simulink model "Problem_3"  (R2020a)
settings: Solver=VariableStepAuto  StartTime=0.0  StopTime=10.0  RelTol=1e-3
settings Model: Creator=Shubham Singh Rathor  LastModifiedBy=Shubham Singh Rathor

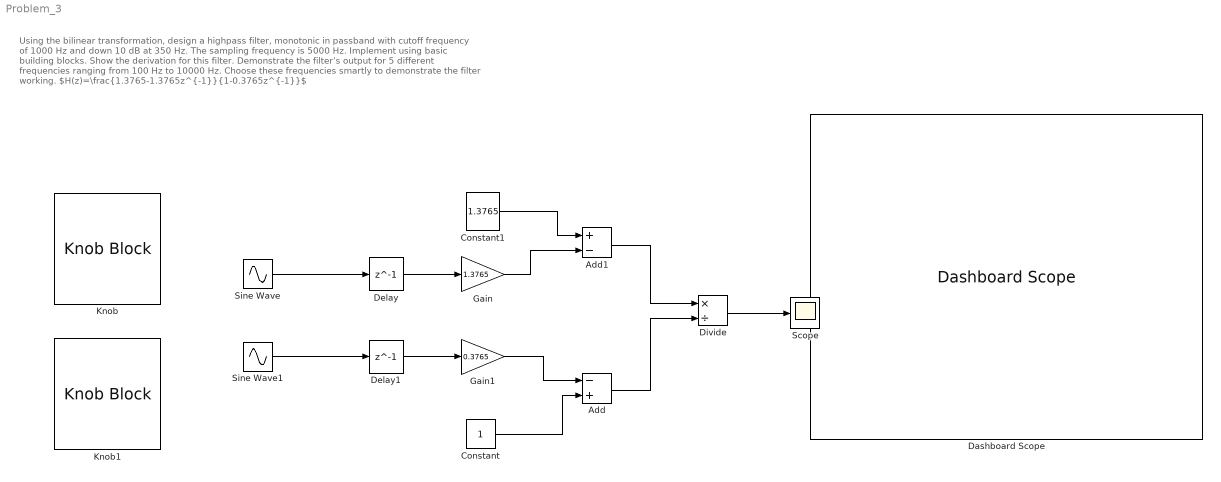
== system Problem_3 ==
  note: Using the bilinear transformation, design a highpass filter, monotonic in passband with cutoff frequency of 1000 Hz and down 10 dB at 350 Hz.
      | The sampling frequency is 5000 Hz. Implement using basic building blocks. Show the derivation for this filter.
      | Demonstrate the filter’s output for 5 different frequencies ranging from 100 Hz to 10000 Hz.
      | Choose these frequencies smartly to demonstrate the filter working.
      | $H(z)=\frac{1.3765-1.3765z^{-1}}{1-0.3765z^{-1}}$
  Add : Sum  Inputs=-+
  Add1 : Sum  Inputs=+-
  Constant : Constant
  Constant1 : Constant  Value=1.3765
  Dashboard Scope : DashboardScope
  Delay : Delay  DelayLength=1
  Delay1 : Delay  DelayLength=1
  Divide : Product  Inputs=*/
  Gain : Gain  Gain=1.3765
  Gain1 : Gain  Gain=0.3765
  Knob : KnobBlock  ScaleMin=100  ScaleMax=10000
  Knob1 : KnobBlock  ScaleMin=100  ScaleMax=10000
  Scope : Scope
  Sine Wave : Sin  Amplitude=2  Frequency=6133.257125854492  SampleTime=0
  Sine Wave1 : Sin  Frequency=5996.515289306641  SampleTime=0
  wires:
  Delay/1 -> Gain/1
  Delay1/1 -> Gain1/1
  Gain1/1 -> Add/1
  Constant/1 -> Add/2
  Constant1/1 -> Add1/1
  Gain/1 -> Add1/2
  Add1/1 -> Divide/1
  Add/1 -> Divide/2
  Divide/1 -> Scope/1
  Sine Wave/1 -> Delay/1
  Sine Wave1/1 -> Delay1/1
